simulink subsystem "OFDM_demodulator"  (R2022a)
settings: Solver=VariableStepAuto  StartTime=0.0  StopTime=10.0  RelTol=1e-3
values from neighbouring files (symbols this model uses):
  cpLength = 20    [initSefdmModel.m]
  frameNum = dataNum + preambleNum    (= 18)    [initSefdmModel.m]
  indiciesWithoutCP = [cpLength+1:issuedSize+cpLength]    [initSefdmModel.m]
  issuedSize = N2*2    (= 508)    [initSefdmModel.m]
libraries: dspxfrm3 x1, dspindex x1
settings Model: Creator=lsfan  LastModifiedBy=lsfan

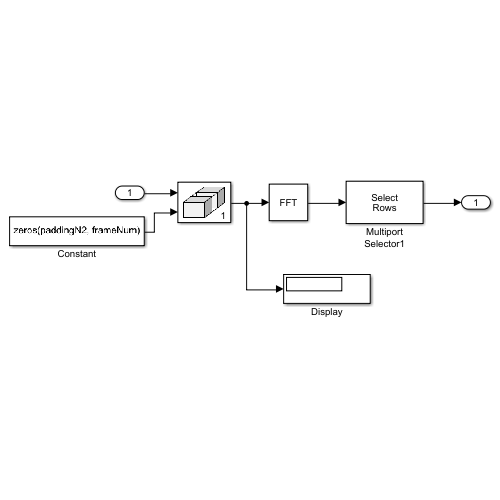
[thumbnail: Simulink's stored preview of the top-level diagram]
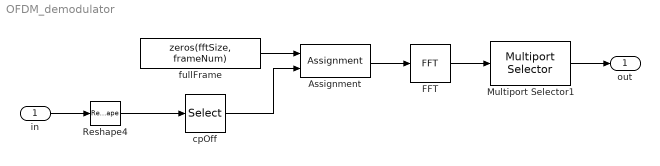
== system OFDM_demodulator ==
  in : Inport
  Assignment : Assignment  NumberOfDimensions=2  DiagnosticForDimensions=Warning  IndexOptions=Index vector (dialog),Assign all  Indices=1:issuedSize,1  OutputSizes=1,1
  FFT : dspxfrm3/FFT  FFTImplementation=Auto  CompMethod=Table lookup  TableOpt=NEW  TableOptActive=Speed  BitRevOrder=off  Normalize=off  InheritFFTLength=on  FFTLength=64  WrapInput=on  roundingMode=Floor  overflowMode=off  firstCoeffDataTypeStr=Inherit: Same word length as input  firstCoeffLastDataTypeStr=Inherit: Same word length as input  outputMin=[]  outputMax=[]
  Multiport Selector1 : dspindex/Multiport Selector  rowsOrCols=Rows  idxCellArray={[channelInUse]}  idxErrMode=Clip Index
  Reshape4 : Reshape  OutputDimensionality=Customize  OutputDimensions=[issuedSize+cpLength, frameNum]
  cpOff : Selector  NumberOfDimensions=2  InputPortWidth=3  IndexOptions=Index vector (dialog),Select all  Indices=indiciesWithoutCP,1  OutputSizes=1,1
  fullFrame : Constant  Value=zeros(fftSize, frameNum)  VectorParams1D=off  SampleTime=-1
  out : Outport
  wires:
  Assignment/1 -> FFT/1
  Reshape4/1 -> cpOff/1
  Multiport Selector1/1 -> out/1
  cpOff/1 -> Assignment/2
  fullFrame/1 -> Assignment/1
  in/1 -> Reshape4/1
  FFT/1 -> Multiport Selector1/1
